simulink model "tresEntradas"  (R2015a)
settings: Solver=ode45  SolverMode=SingleTasking  StartTime=0.0  StopTime=7  RelTol=12e-3
libraries: fuzblock x2, simulink_extras x2, simulink x1
settings Model: CovMetricSettings=dwe  CovHtmlReporting=off  covSaveCumulativeToWorkspaceVar=off  CovSaveSingleToWorkspaceVar=off  CovExternalEMLEnable=on  Creator=brand  LastModifiedBy=brand
settings DataIOCC: LimitDataPoints=off  SaveFormat=Dataset
settings DebuggingCC: SFUnexpectedBacktrackingDiag=error  SFNoUnconditionalDefaultTransitionDiag=error
settings HardwareCC: ProdBitPerPointer=64  ProdLargestAtomicFloat=Float  ProdIntDivRoundTo=Zero  ProdEndianess=LittleEndian  ProdHWDeviceType=Specified
settings ModelReferenceCC: PropagateSignalLabelsOutOfModel=on
settings GRTTargetCC: TargetLangStandard=C99 (ISO)  GeneratePreprocessorConditionals=Use local settings

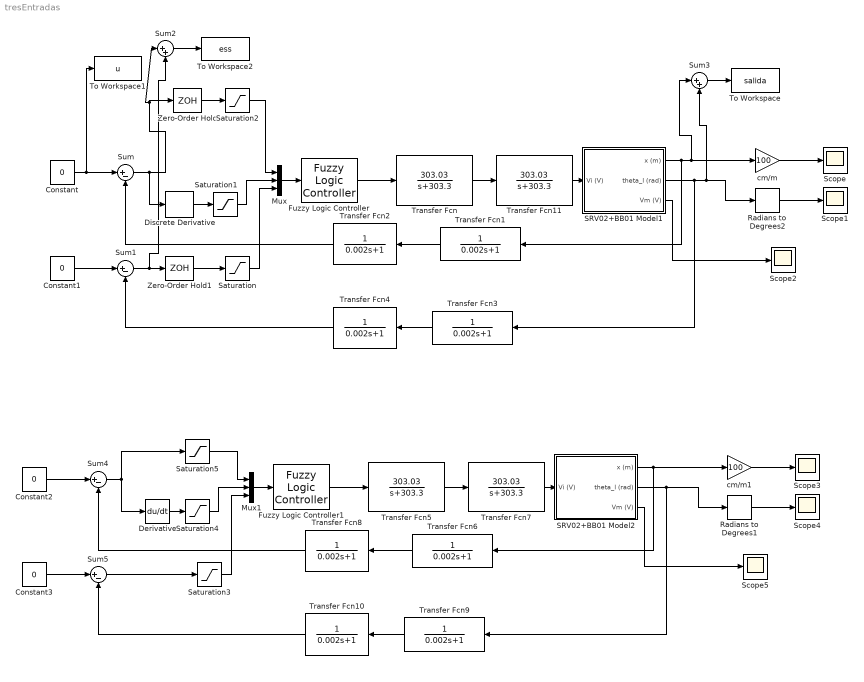
== system tresEntradas ==
  Constant{,1..3} (4 alike) : Constant  Value=0
  Derivative : Derivative
  Discrete Derivative : simulink/Discrete/Discrete Derivative  gainval=1.0  ICPrevScaledInput=0.0  OutMin=[]  OutMax=[]  OutDataType=fixdt(1, 16)  OutScaling=2^-10  DoSatur=off
  Fuzzy Logic Controller : fuzblock/Fuzzy Logic  Controller  FIS=posAngv2unicamf
  Fuzzy Logic Controller1 : fuzblock/Fuzzy Logic  Controller  FIS=posAngv2Opti
  Mux : Mux  Inputs=3
  Mux1 : Mux  Inputs=3
  Radians to Degrees1 : simulink_extras/Transformations/Radians to Degrees
  Radians to Degrees2 : simulink_extras/Transformations/Radians to Degrees
  SRV02+BB01 Model1 : Subsystem
  SRV02+BB01 Model2 : Subsystem
  Saturation : Saturate  UpperLimit=0.785  LowerLimit=-0.785
  Saturation{1..2,4..5} (4 alike) : Saturate  UpperLimit=0.2  LowerLimit=-0.2
  Saturation3 : Saturate  UpperLimit=0.785  LowerLimit=-0.785
  Scope{,1..5} (6 alike) : Scope
      Scope settings: TimeRange=auto  MaxDataPoints=5000  SaveName=difuso  YMin=-2.24341  YMax=5.80482  SampleTime=-1  DataFormat=Array
      Scope1 settings: TimeRange=auto  MaxDataPoints=5000  SaveName=angulo1  YMin=-11.90415  YMax=4.5907  SampleTime=-1  DataFormat=Array
      Scope2 settings: TimeRange=auto  MaxDataPoints=5000  SaveName=difuso1  YMin=-3.16432  YMax=3.13289  SampleTime=-1  DataFormat=Array
      Scope3 settings: TimeRange=auto  MaxDataPoints=5000  SaveName=difuso2  YMin=-4.35501  YMax=6.03945  SampleTime=-1  DataFormat=Array
      Scope4 settings: TimeRange=auto  MaxDataPoints=5000  SaveName=angulo2  YMin=-6.36154  YMax=4.23655  SampleTime=-1  DataFormat=Array
      Scope5 settings: TimeRange=auto  MaxDataPoints=5000  SaveName=difuso3  YMin=-3.16432  YMax=3.13289  SampleTime=-1  DataFormat=Array
  Sum{,1,4..5} (4 alike) : Sum  Inputs=|+-
  Sum2 : Sum  Inputs=|++
  Sum3 : Sum  Inputs=|++
  To Workspace : ToWorkspace  VariableName=salida  SaveFormat=Structure With Time  SampleTime=-1
  To Workspace1 : ToWorkspace  VariableName=u  SampleTime=-1
  To Workspace2 : ToWorkspace  VariableName=ess  SampleTime=-1
  Transfer Fcn{,5,7,11} (4 alike) : TransferFcn  Numerator=[303.03]  Denominator=[1 303.3]
  Transfer Fcn{1..4,6,8..10} (8 alike) : TransferFcn  Denominator=[0.002 1]
  Zero-Order Hold : ZeroOrderHold  SampleTime=12e-3
  Zero-Order Hold1 : ZeroOrderHold  SampleTime=12e-3
  cm/m : Gain  Gain=100
  cm/m1 : Gain  Gain=100
  wires:
  SRV02+BB01 Model1/1(x (m)) -> Transfer Fcn1/1, Sum3/1, cm/m/1
  cm/m/1 -> Scope/1
  Radians to Degrees2/1 -> Scope1/1
  Mux/1 -> Fuzzy Logic Controller/1
  Constant/1 -> To Workspace1/1, Sum/1
  Saturation/1 -> Mux/3
  SRV02+BB01 Model1/2(theta_l (rad)) -> Transfer Fcn3/1, Sum3/2, Radians to Degrees2/1
  Discrete Derivative/1 -> Saturation1/1
  Transfer Fcn/1 -> Transfer Fcn11/1
  Fuzzy Logic Controller/1 -> Transfer Fcn/1
  Transfer Fcn11/1 -> SRV02+BB01 Model1/1(Vi (V))
  Transfer Fcn1/1 -> Transfer Fcn2/1
  Transfer Fcn2/1 -> Sum/2
  Transfer Fcn3/1 -> Transfer Fcn4/1
  Transfer Fcn4/1 -> Sum1/2
  Constant1/1 -> Sum1/1
  Sum1/1 -> Sum2/2, Zero-Order Hold1/1
  Saturation1/1 -> Mux/2
  Saturation2/1 -> Mux/1
  SRV02+BB01 Model1/3(Vm (V)) -> Scope2/1
  Zero-Order Hold/1 -> Saturation2/1
  Sum/1 -> Sum2/1, Zero-Order Hold/1, Discrete Derivative/1
  Zero-Order Hold1/1 -> Saturation/1
  Sum2/1 -> To Workspace2/1
  Sum3/1 -> To Workspace/1
  Sum5/1 -> Saturation3/1
  Sum4/1 -> Derivative/1, Saturation5/1
  SRV02+BB01 Model2/3(Vm (V)) -> Scope5/1
  Saturation5/1 -> Mux1/1
  Saturation4/1 -> Mux1/2
  Constant3/1 -> Sum5/1
  Transfer Fcn10/1 -> Sum5/2
  Transfer Fcn9/1 -> Transfer Fcn10/1
  Transfer Fcn8/1 -> Sum4/2
  Transfer Fcn6/1 -> Transfer Fcn8/1
  Transfer Fcn7/1 -> SRV02+BB01 Model2/1(Vi (V))
  Fuzzy Logic Controller1/1 -> Transfer Fcn5/1
  Transfer Fcn5/1 -> Transfer Fcn7/1
  SRV02+BB01 Model2/2(theta_l (rad)) -> Radians to Degrees1/1, Transfer Fcn9/1
  Saturation3/1 -> Mux1/3
  Constant2/1 -> Sum4/1
  Mux1/1 -> Fuzzy Logic Controller1/1
  Radians to Degrees1/1 -> Scope4/1
  cm/m1/1 -> Scope3/1
  SRV02+BB01 Model2/1(x (m)) -> cm/m1/1, Transfer Fcn6/1
  Derivative/1 -> Saturation4/1

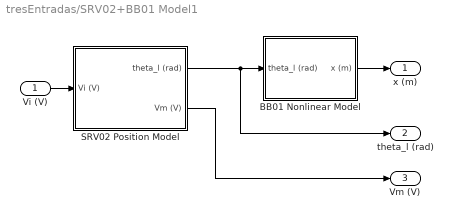
== system tresEntradas/SRV02+BB01 Model1 ==
  Vi (V) : Inport
  BB01 Nonlinear Model : Subsystem
  SRV02 Position Model : Subsystem
  x (m) : Outport
  theta_l (rad) : Outport  Port=2
  Vm (V) : Outport  Port=3
  wires:
  SRV02 Position Model/1(theta_l (rad)) -> BB01 Nonlinear Model/1(theta_l (rad)), theta_l (rad)/1
  BB01 Nonlinear Model/1(x (m)) -> x (m)/1
  Vi (V)/1 -> SRV02 Position Model/1(Vi (V))
  SRV02 Position Model/2(Vm (V)) -> Vm (V)/1

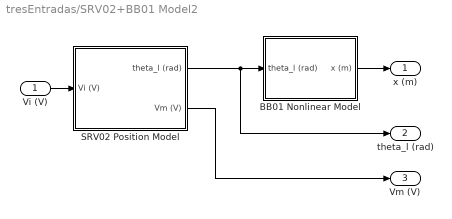
== system tresEntradas/SRV02+BB01 Model2 ==
  Vi (V) : Inport
  BB01 Nonlinear Model : Subsystem
  SRV02 Position Model : Subsystem
  x (m) : Outport
  theta_l (rad) : Outport  Port=2
  Vm (V) : Outport  Port=3
  wires:
  SRV02 Position Model/2(Vm (V)) -> Vm (V)/1
  Vi (V)/1 -> SRV02 Position Model/1(Vi (V))
  BB01 Nonlinear Model/1(x (m)) -> x (m)/1
  SRV02 Position Model/1(theta_l (rad)) -> theta_l (rad)/1, BB01 Nonlinear Model/1(theta_l (rad))

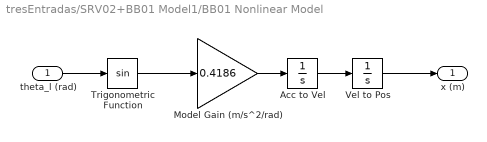
== system tresEntradas/SRV02+BB01 Model1/BB01 Nonlinear Model ==
  theta_l (rad) : Inport
  Acc to Vel : Integrator
  Model Gain (m/s^2/rad) : Gain  Gain=0.4186
  Trigonometric Function : Trigonometry
  Vel to Pos : Integrator  InitialCondition=0.05
  x (m) : Outport
  wires:
  theta_l (rad)/1 -> Trigonometric Function/1
  Vel to Pos/1 -> x (m)/1
  Model Gain (m/s^2/rad)/1 -> Acc to Vel/1
  Acc to Vel/1 -> Vel to Pos/1
  Trigonometric Function/1 -> Model Gain (m/s^2/rad)/1

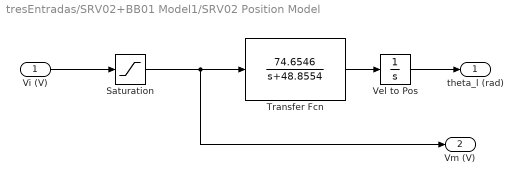
== system tresEntradas/SRV02+BB01 Model1/SRV02 Position Model ==
  Vi (V) : Inport
  Saturation : Saturate  UpperLimit=5  LowerLimit=-5
  Transfer Fcn : TransferFcn  Numerator=[74.6546]  Denominator=[1 48.8554]
  Vel to Pos : Integrator
  theta_l (rad) : Outport
  Vm (V) : Outport  Port=2
  wires:
  Transfer Fcn/1 -> Vel to Pos/1
  Vel to Pos/1 -> theta_l (rad)/1
  Saturation/1 -> Vm (V)/1, Transfer Fcn/1
  Vi (V)/1 -> Saturation/1

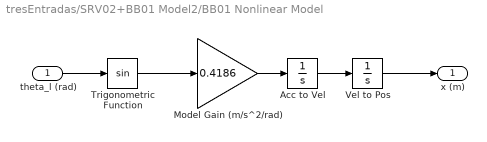
== system tresEntradas/SRV02+BB01 Model2/BB01 Nonlinear Model ==
  theta_l (rad) : Inport
  Acc to Vel : Integrator
  Model Gain (m/s^2/rad) : Gain  Gain=0.4186
  Trigonometric Function : Trigonometry
  Vel to Pos : Integrator  InitialCondition=0.05
  x (m) : Outport
  wires:
  Trigonometric Function/1 -> Model Gain (m/s^2/rad)/1
  Acc to Vel/1 -> Vel to Pos/1
  Model Gain (m/s^2/rad)/1 -> Acc to Vel/1
  Vel to Pos/1 -> x (m)/1
  theta_l (rad)/1 -> Trigonometric Function/1

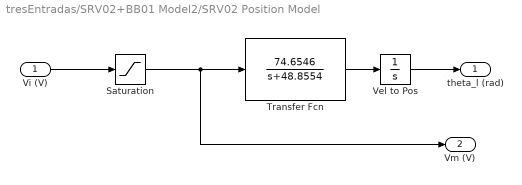
== system tresEntradas/SRV02+BB01 Model2/SRV02 Position Model ==
  Vi (V) : Inport
  Saturation : Saturate  UpperLimit=5  LowerLimit=-5
  Transfer Fcn : TransferFcn  Numerator=[74.6546]  Denominator=[1 48.8554]
  Vel to Pos : Integrator
  theta_l (rad) : Outport
  Vm (V) : Outport  Port=2
  wires:
  Vi (V)/1 -> Saturation/1
  Saturation/1 -> Transfer Fcn/1, Vm (V)/1
  Vel to Pos/1 -> theta_l (rad)/1
  Transfer Fcn/1 -> Vel to Pos/1
